simulink model "fbifwr2"  (R2016a)
settings: Solver=ode23tb  StartTime=0.0  StopTime=0.1  MaxStep=2e-7  RelTol=1e-3  AbsTol=.01
libraries: powerlib x18, simulink x3
settings Model: Creator=Administrator  LastModifiedBy=user
settings DataIOCC: LimitDataPoints=on  SaveFormat=Array  SignalLoggingSaveFormat=ModelDataLogs
settings OptimizationCC: InitFltsAndDblsToZero=on
settings DebuggingCC: SaveWithParameterizedLinksMsg=none  UnderspecifiedInitializationDetection=Classic  MergeDetectMultiDrivingBlocksExec=none  SignalResolutionControl=TryResolveAllWithWarning  SolverPrmCheckMsg=warning  MultiTaskDSMMsg=warning  MultiTaskCondExecSysMsg=none  FcnCallInpInsideContextMsg=EnableAllAsWarning  UnconnectedInputMsg=none  UnconnectedOutputMsg=none  UnconnectedLineMsg=none
settings HardwareCC: ProdBitPerPointer=32  ProdLargestAtomicFloat=None  ProdIntDivRoundTo=Undefined  ProdEndianess=Unspecified  ProdWordSize=32  ProdHWDeviceType=32-bit Generic
settings ModelReferenceCC: PropagateSignalLabelsOutOfModel=off
settings GRTTargetCC: TargetFcnLib=ansi_tfl_tmw.mat  GeneratePreprocessorConditionals=Use local settings  CombineOutputUpdateFcns=off  GRTInterface=on
settings ConfigComp: CovModelRefEnable=Off

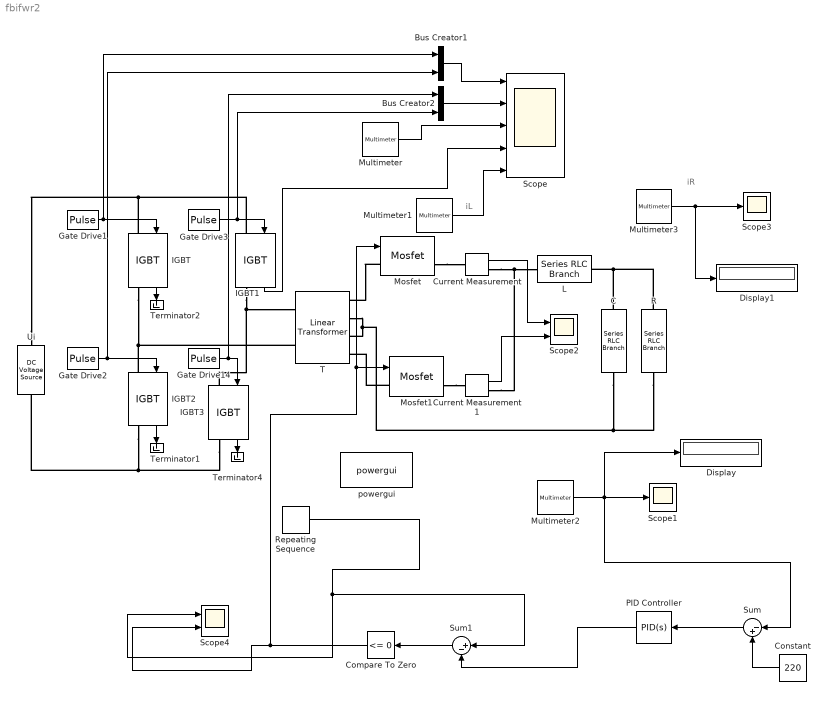
== system fbifwr2 ==
  note: iL
  note: iR
  Bus Creator1 : BusCreator  DialogController=Simulink.DDGSource_Bus  Inputs=2
  Bus Creator2 : BusCreator  DialogController=Simulink.DDGSource_Bus  Inputs=2
  C : powerlib/Elements/Series RLC Branch  LConnTagsString=__new0  RConnTagsString=__new0  BranchType=C  Resistance=0  Inductance=0  SetiL0=off  InitialCurrent=0  Capacitance=3e-4  Setx0=off  InitialVoltage=0  Measurements=None
  Compare To Zero : simulink/Logic and Bit Operations/Compare To Zero  relop=<=  OutDataTypeStr=boolean
  Constant : Constant  Value=220
  Current Measurement : powerlib/Measurements/Current Measurement  PhasorSimulation=off  OutputType=Complex  PSBequivalent=0
  Current Measurement1 : powerlib/Measurements/Current Measurement  PhasorSimulation=off  OutputType=Complex  PSBequivalent=0
  Display : Display
  Display1 : Display
  Gate Drive1 : DiscretePulseGenerator  PulseType=Time based  Period=5e-5  PulseWidth=25
  Gate Drive14 : DiscretePulseGenerator  PulseType=Time based  Period=5e-5  PulseWidth=25
  Gate Drive2 : DiscretePulseGenerator  PulseType=Time based  Period=5e-5  PulseWidth=25  PhaseDelay=180/7200000
  Gate Drive3 : DiscretePulseGenerator  PulseType=Time based  Period=5e-5  PulseWidth=25  PhaseDelay=180/7200000
  IGBT{,1..3} (4 alike) : powerlib/Power Electronics/IGBT  Ron=0  Lon=0  Vf=0  Tf=1e-6  Tt=2e-6  IC=0  Rs=inf  Cs=inf  Measurements=on
  L : powerlib/Elements/Series RLC Branch  LConnTagsString=__new0  RConnTagsString=__new0  BranchType=L  Resistance=0  Inductance=5e-3  SetiL0=off  InitialCurrent=0  Capacitance=inf  Setx0=off  InitialVoltage=0  Measurements=Branch voltage and current
  Mosfet : powerlib/Power Electronics/Mosfet  Ron=1  Lon=0  Rd=0.0001  Vfd=0  IC=0  Rs=1e5  Cs=inf  Measurements=on
  Mosfet1 : powerlib/Power Electronics/Mosfet  Ron=1  Lon=0  Rd=0.0001  Vfd=0  IC=0  Rs=1e5  Cs=inf  Measurements=on
  Multimeter : powerlib/Measurements/Multimeter  PhasorSimulation=off  OutputType=Complex  sel=[3 8]  L=13  Gain=[1 1]  yselected={'Uw1: T','Iw1: T'};  PSBOutputType=1  PSBequivalent=0  AxesSetting=[0,0.1,-100,100]  Display=0  SavedBlockNames=-11
  Multimeter1 : powerlib/Measurements/Multimeter  PhasorSimulation=off  OutputType=Complex  sel=6  L=13  Gain=1  yselected={'Ib: L'};  PSBOutputType=1  PSBequivalent=0  AxesSetting=[0,0.1,-100,100]  Display=0  SavedBlockNames=-11
  Multimeter2 : powerlib/Measurements/Multimeter  PhasorSimulation=off  OutputType=Complex  sel=2  L=13  Gain=-1  yselected={'Ub: R'};  PSBOutputType=1  PSBequivalent=0  AxesSetting=[0,0.1,-100,100]  Display=0  SavedBlockNames=-11
  Multimeter3 : powerlib/Measurements/Multimeter  PhasorSimulation=off  OutputType=Complex  sel=7  L=13  Gain=-1  yselected={'Ib: R'};  PSBOutputType=1  PSBequivalent=0  AxesSetting=[0,0.1,-100,100]  Display=0  SavedBlockNames=-11
  PID Controller : simulink/Continuous/PID Controller  Controller=PID  TimeDomain=Continuous-time  SampleTime=-1  IntegratorMethod=Forward Euler  FilterMethod=Forward Euler  Form=Parallel  UseFilter=on  ControllerParametersSource=internal  P=1  I=10  D=10  N=100  InitialConditionSource=internal  InitialConditionForIntegrator=0  InitialConditionForFilter=0  ExternalReset=none  LimitOutput=off  UpperSaturationLimit=inf  LowerSaturationLimit=-inf  LinearizeAsGain=on  AntiWindupMode=none  Kb=1  TrackingMode=off  Kt=1  PParamMin=[]  PParamMax=[]  IParamMin=[]  IParamMax=[]  DParamMin=[]  DParamMax=[]  NParamMin=[]  NParamMax=[]  KbParamMin=[]  KbParamMax=[]  KtParamMin=[]  KtParamMax=[]  POutMin=[]  POutMax=[]  IOutMin=[]  IOutMax=[]  DOutMin=[]  DOutMax=[]  NOutMin=[]  NOutMax=[]  KbOutMin=[]  KbOutMax=[]  KtOutMin=[]  KtOutMax=[]  IntegratorOutMin=[]  IntegratorOutMax=[]  FilterOutMin=[]  FilterOutMax=[]  SumOutMin=[]  SumOutMax=[]  SumI1OutMin=[]  SumI1OutMax=[]  SumI2OutMin=[]  SumI2OutMax=[]  SumI3OutMin=[]  SumI3OutMax=[]  SumDOutMin=[]  SumDOutMax=[]  SaturationOutMin=[]  SaturationOutMax=[]  IntegratorContinuousStateAttributes=''  IntegratorStateMustResolveToSignalObject=off  IntegratorRTWStateStorageClass=Auto  FilterContinuousStateAttributes=''  FilterStateMustResolveToSignalObject=off  FilterRTWStateStorageClass=Auto  DifferentiatorICPrevScaledInput=0  DifferentiatorOutMin=[]  DifferentiatorOutMax=[]
  R : powerlib/Elements/Series RLC Branch  LConnTagsString=__new0  RConnTagsString=__new0  BranchType=R  Resistance=220/30  Inductance=0  SetiL0=off  InitialCurrent=0  Capacitance=inf  Setx0=off  InitialVoltage=0  Measurements=Branch voltage and current
  Repeating Sequence : simulink/Sources/Repeating Sequence  rep_seq_t=[0 1/800000]  rep_seq_y=[0 2]
  Scope : Scope  NumInputPorts=5
  Scope1 : Scope
  Scope2 : Scope  NumInputPorts=2
  Scope3 : Scope
  Scope4 : Scope  NumInputPorts=2
  Sum : Sum  Inputs=|-+
  Sum1 : Sum  Inputs=|+-
  T : powerlib/Elements/Linear Transformer  UNITS=pu  NominalPower=[500 20000 ]  winding1=[300 0 0]  winding2=[11000 0 0]  ThreeWindings=on  winding3=[11000 0 0]  RmLm=[inf inf]  Measurements=All voltages and currents  DataType=off
  Terminator1 : Terminator
  Terminator2 : Terminator
  Terminator4 : Terminator
  Ui : powerlib/Electrical Sources/DC Voltage Source  Amplitude=12  Measurements=None
  powergui : powerlib/powergui  Priority=1  SimulationMode=Continuous  SolverType=Tustin/Backward Euler (TBE)  SampleTime=50e-6  frequency=60  SPID=on  DisableSnubberDevices=off  DisableRonSwitches=off  DisableVfSwitches=off  SwTol=0  DisplayEquations=off  Interpol=off  ExternalGateDelay=off  methode=off  Ts=100  FunctionMessages=off  echomessages=off  HookPort=off  EnableUseOfTLC=off  x0status=blocks  frequencyindice=0  Pbase=100e6  ErrMax=1e-4  Iterations=50  UnitsV=kV  UnitsW=MW  buscounter=0  RestoreLinks=warning  ResistiveCurrentMeasurement=off  Frange=[0:2:500]  Ylog=off  Xlog=on  ShowGrid=off  save=off  variable=ZData  structure=0  ZoomFFT=off  StartTime=0.0  cycles=1  DisplayStyle=1  fundamental=60  FreqAxis=off  MaxFrequency=1000  frequencyindicesteady=1  RmsSteady=1  display=off
  wires:
  Gate Drive1/1 -> IGBT/1, Bus Creator1/1
  Multimeter/1 -> Scope/3
  Gate Drive2/1 -> IGBT2/1, Bus Creator1/2
  IGBT2/1 -> Terminator1/1
  IGBT3/1 -> Terminator4/1
  Gate Drive3/1 -> IGBT1/1, Bus Creator2/2
  Gate Drive14/1 -> IGBT3/1, Bus Creator2/1
  Bus Creator1/1 -> Scope/1
  Bus Creator2/1 -> Scope/2
  IGBT1/1 -> Scope/4
  Multimeter1/1 -> Scope/5
  Current Measurement/1 -> Scope2/1
  Current Measurement1/1 -> Scope2/2
  Multimeter3/1 -> Scope3/1, Display1/1
  IGBT/1 -> Terminator2/1
  Constant/1 -> Sum/2
  Multimeter2/1 -> Sum/1, Display/1, Scope1/1
  Sum/1 -> PID Controller/1
  Repeating Sequence/1 -> Sum1/1, Scope4/1
  Sum1/1 -> Compare To Zero/1
  PID Controller/1 -> Sum1/2
  Compare To Zero/1 -> Scope4/2, Mosfet/1, Mosfet1/1
  connections:
  IGBT3/RConn1 -- Ui/LConn1 -- IGBT2/RConn1
  IGBT1/RConn1 -- T/LConn1 -- IGBT3/LConn1
  T/LConn2 -- IGBT2/LConn1 -- IGBT/RConn1
  Mosfet/LConn1 -- T/RConn1
  C/LConn1 -- L/RConn1 -- R/LConn1
  Current Measurement/RConn1 -- Current Measurement1/RConn1 -- L/LConn1
  R/RConn1 -- C/RConn1 -- T/RConn2 -- T/RConn3
  Mosfet1/LConn1 -- T/RConn4
  Ui/RConn1 -- IGBT1/LConn1 -- IGBT/LConn1
  Mosfet/RConn1 -- Current Measurement/LConn1
  Mosfet1/RConn1 -- Current Measurement1/LConn1
